simulink model "TFlex_I_FITC"  (R2018a)
settings: Solver=VariableStepAuto  StartTime=0.0  StopTime=10.0  RelTol=1e-3
undefined symbols (not defined in the file): a0, a1, a2, Avout, b, D, DiscIntNeverNeededParam, FB1_offset, h, hyp, I_limit_max, I_limit_min, Kd, Ki, Kp, kp, KTY_p0, KTY_p1, Kuu, LPden, LPnum, Lu, mu_u, Nkeep, R, r, seed, sf, SIGMA, sn, sp_ts, tau_i, tau_p, tau_z, tm, ts, var_u, w
libraries: xpcethercatlib x17, simulink x10, dspindex x6, slrtlib x5, dspfactors x2, dspmtrx3 x2
(part 1 of 2)
settings Model: Creator=wout7  LastModifiedBy=wout7

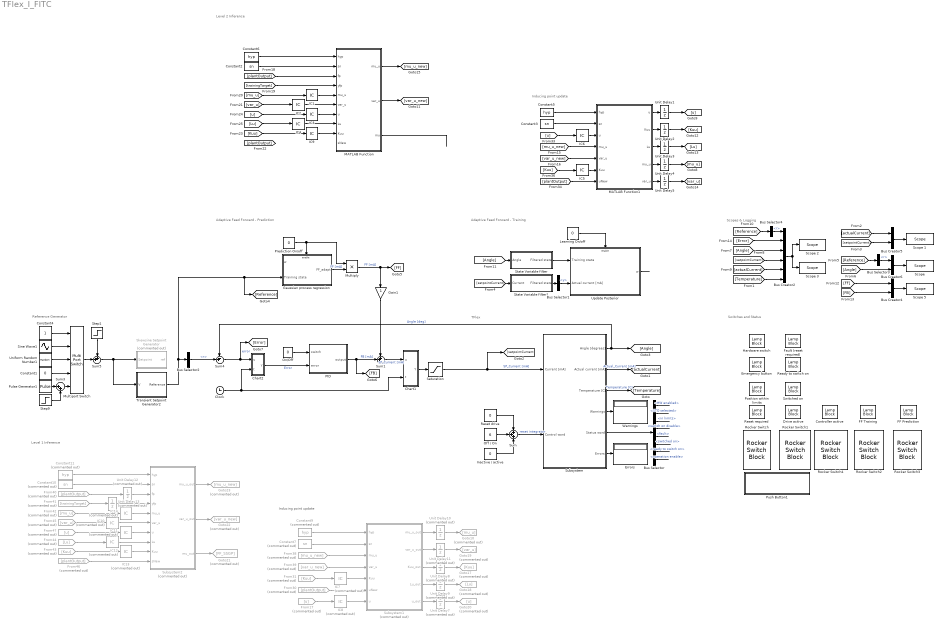
== system TFlex_I_FITC ==
  note: Switches and Status
  note: Adaptive Feed Forward - Prediction
  note: TFlex
  note: Scopes & Logging
  note: Reference Generator
  note: Adaptive Feed Forward - Training
  note: Inducing point update
  note: Inducing point update
  note: Level 2 Inference
  note: Level 1 Inference
  Bus Creator2 : BusCreator  Inputs=6
  Bus Creator4 : BusCreator  Inputs=2
  Bus Creator5 : BusCreator  Inputs=2
  Bus Creator6 : BusCreator  Inputs=2
  Bus Selector : BusSelector  OutputSignals=HW enabled,STO selected,in limits,switch on disable,fault,switched on,ready to switch on,operation enable
  Bus Selector1 : BusSelector  OutputSignals=y
  Bus Selector2 : BusSelector  OutputSignals=r
  Bus Selector3 : BusSelector  OutputSignals=r
  Bus Selector4 : BusSelector  OutputSignals=r
  Chart1 : Stateflow chart  TreatAsAtomicUnit=on
  Chart2 : Stateflow chart  TreatAsAtomicUnit=on
  Clock : Clock
  Constant1 : Constant  Value=0  SampleTime=sp_ts
  Constant10 : Constant  Commented=on  Value=sn  SampleTime=-1
  Constant11 : Constant  Commented=on  Value=hyp  SampleTime=-1
  Constant2 : Constant  Value=sn  SampleTime=-1
  Constant3 : Constant  Value=sn  SampleTime=-1
  Constant4 : Constant  SampleTime=sp_ts
  Constant5 : Constant  Value=hyp  SampleTime=-1
  Constant6 : Constant  Value=hyp  SampleTime=-1
  Constant7 : Constant  Commented=on  Value=sn  SampleTime=-1
  Constant9 : Constant  Commented=on  Value=hyp  SampleTime=-1
  Controller active : LampBlock  WebBlockId=392  LabelPosition=Hide
  Drive active : LampBlock  WebBlockId=394
  Emergency button : LampBlock  WebBlockId=395
  Errors : Display
  FF Prediction : LampBlock  WebBlockId=397  LabelPosition=Hide
  FF Training : LampBlock  WebBlockId=398  LabelPosition=Hide
  Fault (reset required) : LampBlock  WebBlockId=399
  From17 : From  Commented=on  GotoTag=u
  From30 : From  Commented=on  GotoTag=plantOutput
  From31 : From  Commented=on  GotoTag=Kuu
  From38 : From  Commented=on  GotoTag=mu_u_new
  From39 : From  Commented=on  GotoTag=var_u_new
  From40 : From  Commented=on  GotoTag=plantOutput
  From41 : From  Commented=on  GotoTag=trainingTarget
  From42 : From  Commented=on  GotoTag=mu_u
  From43 : From  Commented=on  GotoTag=Kuu
  From44 : From  Commented=on  GotoTag=Lu
  From45 : From  Commented=on  GotoTag=var_u
  From46 : From  Commented=on  GotoTag=plantOutput
  From47 : From  Commented=on  GotoTag=u
  Gain1 : Gain
  Gaussian process regression : Subsystem
  Goto10 : Goto  Commented=on  GotoTag=mu_u
  Goto17 : Goto  Commented=on  GotoTag=Kuu
  Goto18 : Goto  Commented=on  GotoTag=Lu
  Goto19 : Goto  Commented=on  GotoTag=var_u
  Goto20 : Goto  Commented=on  GotoTag=u
  Goto21 : Goto  Commented=on  GotoTag=FF_SSGP
  Goto22 : Goto  Commented=on  GotoTag=var_u_new
  Goto23 : Goto  Commented=on  GotoTag=mu_u_new
  Hardware switch : LampBlock  WebBlockId=462
  IC1 : InitialCondition  Value=mu_u
  IC10 : InitialCondition  Commented=on  Value=var_u
  IC11 : InitialCondition  Commented=on  Value=u
  IC12 : InitialCondition  Commented=on  Value=Lu
  IC13 : InitialCondition  Commented=on  Value=Kuu
  IC14 : InitialCondition  Commented=on  Value=mu_u
  IC2 : InitialCondition  Value=var_u
  IC3 : InitialCondition  Value=u
  IC4 : InitialCondition  Value=Lu
  IC5 : InitialCondition  Value=Kuu
  IC6 : InitialCondition  Value=u
  IC7 : InitialCondition  Commented=on  Value=Kuu
  IC8 : InitialCondition  Commented=on  Value=u
  IC9 : InitialCondition  Value=Kuu
  Inactive / active : Constant  Value=0
  Learning On/off : Constant  Value=0
  MATLAB Function : MATLAB Function  TreatAsAtomicUnit=on
  MATLAB Function1 : MATLAB Function  TreatAsAtomicUnit=on
  Multiply : Product
  Multiport Switch : MultiPortSwitch  Inputs=4
  Off / On : Constant  Value=6
  On/Off : Constant  Value=0
  "PID " : Subsystem
  Position within limits : LampBlock  WebBlockId=527
  Prediction On/off : Constant  Value=0  SampleTime=ts
  Pulse Generator1 : DiscretePulseGenerator  Amplitude=46  SampleTime=sp_ts
  Push Button1 : Subsystem  DialogController=hmiCreateDDGDialog  IsWebBlock=on  mask(MWDashboardBlock){webBlockId=a54107f9-bd11-456c-ac83-5802f3df51ad, webBlockType=pushbutton, ShowInLibBrwoser=on, ShowInitialText=on, HMISrcModelName=TFlex_I_FITC}
      mask prompts: webBlockId "WebBlock Id"; webBlockType "WebBlock Type"; HMISrcModelName "Source Model"
      mask help: SimulinkHMI:dialogs:PushButtonDialogDesc
      mask Help: helpview([docroot '/mapfiles/simulink.map'], 'hmi_push_button')
      mask Display:
      | model = bdroot(gcb);
      | if strcmp(get_param(model,'BlockDiagramType'), 'library')
      |     image([(matlabroot) '/toolbox/simulink/hmi/icons/PushButton.png']);
      | end
  Ready to switch on : LampBlock  WebBlockId=531
  Reset drive : Constant  Value=0
  Reset required : LampBlock  WebBlockId=533
  Rocker Switch : RockerSwitchBlock  WebBlockId=534  LabelPosition=Hide
      settings: Values={{'Off', 'Driver On'}, [6 7]}
  Rocker Switch1 : RockerSwitchBlock  WebBlockId=535  LabelPosition=Hide
      settings: Values={{'Inactive', 'Driver Active'}, [0 8]}
  Rocker Switch2 : RockerSwitchBlock  WebBlockId=536  LabelPosition=Hide
      settings: Values={{'Off', 'Training on'}, [0 1]}
  Rocker Switch3 : RockerSwitchBlock  WebBlockId=537  LabelPosition=Hide
      settings: Values={{'Off', 'Prediction On'}, [0 1]}
  Rocker Switch4 : RockerSwitchBlock  WebBlockId=538  LabelPosition=Hide
      settings: Values={{'Off', 'Controller On'}, [0 1]}
  Saturation : Saturate  UpperLimit=750  LowerLimit=-250/2
  "Scope " : slrtlib/Displays and Logging/Scope   scopeno=1  scopetype=Target  autostart=on  viewmode=Graphical redraw  formatstr='%15.6f'  grid=on  ylimits=[0 ,0]  nosamples=2000  noprepostsamples=0  interleave=1  triggermode=FreeRun  triggersignal=1  trigsignalfromport=off  triggerlevel=0.0  triggerslope=Either  triggerscope=1  triggersample=0  filename=data.dat  mode=Lazy  writesize=512  autorestart=off  dynamicfilemode=off  maxwritefilesize=512*1024^2
  Scope 1 : slrtlib/Displays and Logging/Scope   scopeno=2  scopetype=Target  autostart=on  viewmode=Graphical redraw  formatstr='%15.6f'  grid=on  ylimits=[500,500]  nosamples=250  noprepostsamples=0  interleave=1  triggermode=FreeRun  triggersignal=1  trigsignalfromport=off  triggerlevel=0.0  triggerslope=Either  triggerscope=1  triggersample=0  filename=data.dat  mode=Lazy  writesize=512  autorestart=off  dynamicfilemode=off  maxwritefilesize=512*1024^2
  Scope 2 : slrtlib/Displays and Logging/Scope   scopeno=3  scopetype=Target  autostart=on  viewmode=Numerical  formatstr='%15.6f,%15.6f,%15.6f,%15.0f'  grid=on  ylimits=[500,500]  nosamples=250  noprepostsamples=0  interleave=1  triggermode=FreeRun  triggersignal=1  trigsignalfromport=off  triggerlevel=0.0  triggerslope=Either  triggerscope=1  triggersample=0  filename=data.dat  mode=Lazy  writesize=512  autorestart=off  dynamicfilemode=off  maxwritefilesize=512*1024^2
  Scope 3 : slrtlib/Displays and Logging/Scope   scopeno=4  scopetype=File  autostart=on  viewmode=Graphical redraw  formatstr='%15.6f'  grid=on  ylimits=[0,0]  nosamples=600000  noprepostsamples=0  interleave=1  triggermode=FreeRun  triggersignal=1  trigsignalfromport=off  triggerlevel=0.0  triggerslope=Either  triggerscope=1  triggersample=0  filename=data.dat  mode=Lazy  writesize=512  autorestart=off  dynamicfilemode=off  maxwritefilesize=512*1024^2
  Scope 5 : slrtlib/Displays and Logging/Scope   scopeno=5  scopetype=Target  autostart=on  viewmode=Graphical redraw  formatstr='%15.6f'  grid=on  ylimits=[500,500]  nosamples=250  noprepostsamples=0  interleave=1  triggermode=FreeRun  triggersignal=1  trigsignalfromport=off  triggerlevel=0.0  triggerslope=Either  triggerscope=1  triggersample=0  filename=data.dat  mode=Lazy  writesize=512  autorestart=off  dynamicfilemode=off  maxwritefilesize=512*1024^2
  Sine Wave1 : Sin  Amplitude=15  Frequency=2*pi*2  SampleTime=0
  Skewsine Setpoint Generator : Subsystem  Commented=on
  State Variable filter : Subsystem
  State Variable filter1 : Subsystem
  Step1 : Step  Time=20  Before=-23  After=0  SampleTime=0
  Step9 : Step  Time=0  After=-24  SampleTime=sp_ts
  Subsystem : Subsystem
  Subsystem1 : Subsystem  Commented=on
  Subsystem2 : Subsystem  Commented=on
  Sum : Sum  Inputs=+++
  Sum1 : Sum  Inputs=++|
  Sum3 : Sum  Inputs=|++
  Sum4 : Sum  Inputs=-+|
  Sum5 : Sum  Inputs=++|
  Switched on : LampBlock  WebBlockId=680
  Transient Setpoint Generator2 : Subsystem
  Uniform Random Number1 : UniformRandomNumber  Seed=seed  SampleTime=sp_ts
  Unit Delay{1..5} (5 alike) : UnitDelay  SampleTime=-1
  Unit Delay{7..13} (7 alike) : UnitDelay  Commented=on  SampleTime=-1
  Update Posterior : Subsystem
  Warnings : Display
  wires:
  Bus Selector/5 -> ?  "<fault>"
  Bus Selector/8 -> ?  "<operation enable>"
  Bus Selector/7 -> ?  "<ready to switch on>"
  Bus Selector/3 -> ?  "<in limits>"
  Update Posterior/1(w) -> ?
  Subsystem/5(Status word) -> Bus Selector/1
  ? -> Gaussian process regression/1(w)
  Subsystem/1(Angle [degrees]) -> [Angle], Sum4/1  "Angle [deg]"
  Subsystem/6(Errors) -> Errors/1
  Subsystem/2(Actual current [mA]) -> [actualCurrent]  "Actual_Current [mA]"
  Pulse Generator1/1 -> Sum3/1
  Bus Selector/1 -> ?  "<HW enabled>"
  Step9/1 -> Sum3/2
  Gaussian process regression/1(FF_adapt) -> Multiply/2  "FF [mA]"
  [FB] -> Bus Creator4/2
  State Variable filter/1(Filtered state) -> Update Posterior/1(Training state)
  Reset drive/1 -> Sum/1
  Sum3/1 -> Multiport Switch/5
  Constant1/1 -> Multiport Switch/4
  Bus Selector/2 -> ?  "<STO selected>"
  Multiply/1 -> Gain1/1, [FF]  "FF [mA]"
  Bus Selector3/1 -> Bus Creator6/1  "<r>"
  Step1/1 -> Sum5/1
  Bus Creator6/1 -> "Scope "/1
  Saturation/1 -> [setpointCurrent], Subsystem/1(Current [mA])  "SP_Current [mA]"
  Subsystem/3(Temperature [C]) -> [Temperature]  "Temperature [C]"
  Sum/1 -> Subsystem/2(Control word)  "reset integrator"
  Bus Selector4/1 -> Bus Creator2/1  "<r>"
  Chart2/1(Y) -> "PID "/2(error)  "Error"
  Bus Creator5/1 -> Scope 1/1
  [Error] -> Bus Creator2/2
  [setpointCurrent] -> Bus Creator2/4
  Bus Creator4/1 -> Scope 5/1
  State Variable filter1/1(Filtered state) -> Bus Selector1/1
  Bus Selector/4 -> ?  "<switch on disable>"
  [Angle] -> Bus Creator6/2
  Chart1/1(Y) -> Saturation/1
  "PID "/1(output) -> [FB], Sum1/2  "FB [mA]"
  [FF] -> Bus Creator4/1
  [setpointCurrent] -> State Variable filter1/1(Current)
  [actualCurrent] -> Bus Creator5/1
  Sine Wave1/1 -> Multiport Switch/2
  [actualCurrent] -> Bus Creator2/5
  Subsystem/4(Warnings) -> Warnings/1
  [setpointCurrent] -> Bus Creator5/2
  Gain1/1 -> Sum1/1
  Sum1/1 -> Chart1/1(u)  "SP_Current [mA]"
  [Reference] -> Bus Selector3/1
  [Temperature] -> Bus Creator2/6
  Sum5/1 -> Skewsine Setpoint Generator/1(Setpoint), Transient Setpoint Generator2/1(V)
  [Reference] -> Bus Selector4/1
  Bus Selector2/1 -> Sum4/2  "<r>"
  Bus Selector1/1 -> Update Posterior/2("Actual current [mA] ")  "<y>"
  Inactive / active/1 -> Sum/3
  [Angle] -> State Variable filter/1(Angle)
  Uniform Random Number1/1 -> Multiport Switch/3
  Bus Creator2/1 -> Scope 2/1, Scope 3/1
  Prediction On/off/1 -> Gaussian process regression/Enable, Multiply/1
  Multiport Switch/1 -> Sum5/2
  Clock/1 -> Chart2/2(t), Chart1/2(t)
  Transient Setpoint Generator2/1(Reference) -> Gaussian process regression/2(Training state), [Reference], Bus Selector2/1
  Sum4/1 -> [Error], Chart2/1(u)  "error"
  Learning On/off/1 -> Update Posterior/Enable
  [Angle] -> Bus Creator2/3
  Off / On/1 -> Sum/2
  Constant4/1 -> Multiport Switch/1
  Bus Selector/6 -> ?  "<switched on>"
  On/Off/1 -> "PID "/1(switch)
  Constant3/1 -> MATLAB Function1/2(sn)
  MATLAB Function1/4(mu_u) -> Unit Delay4/1
  [u] -> IC6/1
  [plantOutput] -> MATLAB Function1/7(uNew)
  [Kuu] -> IC5/1
  IC6/1 -> MATLAB Function1/3("u ")
  Unit Delay3/1 -> [Lu]
  [var_u_new] -> MATLAB Function1/5("var_u ")
  MATLAB Function1/5(var_u) -> Unit Delay5/1
  Constant5/1 -> MATLAB Function1/1(hyp)
  Unit Delay4/1 -> [mu_u]
  MATLAB Function1/2(Kuu) -> Unit Delay2/1
  [mu_u_new] -> MATLAB Function1/4("mu_u ")
  MATLAB Function1/1(u) -> Unit Delay1/1
  IC5/1 -> MATLAB Function1/6("Kuu ")
  Unit Delay5/1 -> [var_u]
  MATLAB Function1/3(Lu) -> Unit Delay3/1
  Unit Delay1/1 -> [u]
  Unit Delay2/1 -> [Kuu]
  Unit Delay9/1 -> Goto18/1
  From31/1 -> IC7/1
  Unit Delay7/1 -> Goto20/1
  Subsystem1/5(u_out) -> Unit Delay7/1
  From17/1 -> IC8/1
  From39/1 -> Subsystem1/4(var_u)
  IC7/1 -> Subsystem1/5(Kuu)
  From38/1 -> Subsystem1/3(mu_u)
  Subsystem1/4(Lu_out) -> Unit Delay9/1
  Subsystem1/3(Kuu_out) -> Unit Delay8/1
  Unit Delay11/1 -> Goto19/1
  Constant9/1 -> Subsystem1/1(hyp)
  Subsystem1/2(var_u_out) -> Unit Delay11/1
  Unit Delay10/1 -> Goto10/1
  From30/1 -> Subsystem1/6(uNew)
  Unit Delay8/1 -> Goto17/1
  Constant7/1 -> Subsystem1/2(sn)
  Subsystem1/1(mu_u_out) -> Unit Delay10/1
  IC8/1 -> Subsystem1/7(u)
  [plantOutput] -> MATLAB Function/3(fp)
  [trainingTarget] -> MATLAB Function/4(yfp)
  IC4/1 -> MATLAB Function/8(Lu)
  IC1/1 -> MATLAB Function/5("mu_u ")
  [Kuu] -> IC9/1
  [var_u] -> IC2/1
  [u] -> IC3/1
  [Lu] -> IC4/1
  Constant2/1 -> MATLAB Function/2(sn)
  [mu_u] -> IC1/1
  IC9/1 -> MATLAB Function/9(Kuu)
  MATLAB Function/1(mu_u) -> [mu_u_new]
  ? -> MATLAB Function/10(sNew)
  MATLAB Function/2(var_u) -> [var_u_new]
  IC2/1 -> MATLAB Function/6("var_u ")
  IC3/1 -> MATLAB Function/7(u)
  Constant6/1 -> MATLAB Function/1(hyp)
  MATLAB Function/3(mu) -> ?
  From44/1 -> IC12/1
  From47/1 -> IC11/1
  Constant11/1 -> Subsystem2/1(hyp)
  Subsystem2/2(var_u_out) -> Goto22/1
  IC12/1 -> Subsystem2/8(Lu)
  Unit Delay12/1 -> Subsystem2/3(fp)
  IC11/1 -> Subsystem2/7(u)
  IC13/1 -> Subsystem2/9(Kuu)
  Unit Delay13/1 -> Subsystem2/4(yfp)
  From40/1 -> Unit Delay12/1
  IC14/1 -> Subsystem2/5(mu_u)
  From46/1 -> Subsystem2/10(sNew)
  Subsystem2/3(mu_out) -> Goto21/1
  From43/1 -> IC13/1
  Subsystem2/1(mu_u_out) -> Goto23/1
  From45/1 -> IC10/1
  From42/1 -> IC14/1
  From41/1 -> Unit Delay13/1
  Constant10/1 -> Subsystem2/2(sn)
  IC10/1 -> Subsystem2/6(var_u)

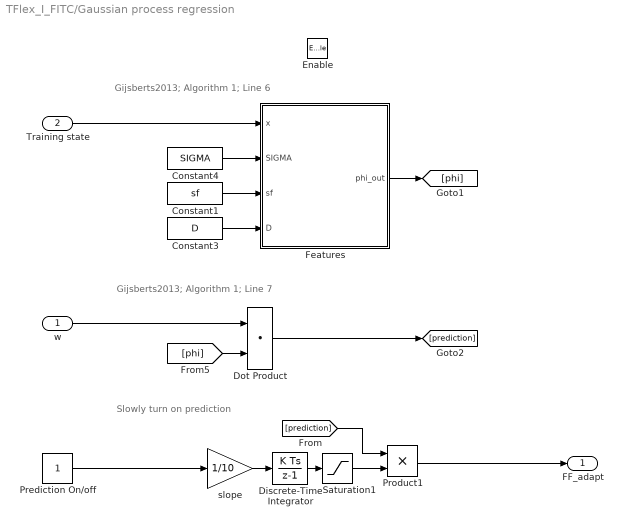
== system TFlex_I_FITC/Gaussian process regression ==
  note: Gijsberts2013; Algorithm 1; Line 7
  note: Gijsberts2013; Algorithm 1; Line 6
  note: Slowly turn on prediction
  w : Inport
  Training state : Inport  Port=2
  Enable : EnablePort  StatesWhenEnabling=reset
  Constant1 : Constant  Value=sf  VectorParams1D=off
  Constant3 : Constant  Value=D  VectorParams1D=off
  Constant4 : Constant  Value=SIGMA  VectorParams1D=off
  Discrete-Time Integrator : DiscreteIntegrator  SampleTime=-1  ICPrevOutput=DiscIntNeverNeededParam  ICPrevScaledInput=DiscIntNeverNeededParam
  Dot Product : DotProduct  OutDataTypeStr=Inherit: Inherit via internal rule
  Features : Subsystem
  Prediction On/off : Constant
  Product1 : Product
  Saturation1 : Saturate  UpperLimit=1  LowerLimit=0
  slope : Gain  Gain=1/10
  FF_adapt : Outport  SampleTime=ts
  wires:
  w/1 -> Dot Product/1
  [phi] -> Dot Product/2
  Product1/1 -> FF_adapt/1
  slope/1 -> Discrete-Time Integrator/1
  Prediction On/off/1 -> slope/1
  Discrete-Time Integrator/1 -> Saturation1/1
  Dot Product/1 -> [prediction]
  Constant4/1 -> Features/2(SIGMA)
  Training state/1 -> Features/1(x)
  Features/1(phi_out) -> [phi]
  Constant3/1 -> Features/4(D)
  Constant1/1 -> Features/3(sf)
  Saturation1/1 -> Product1/2
  [prediction] -> Product1/1

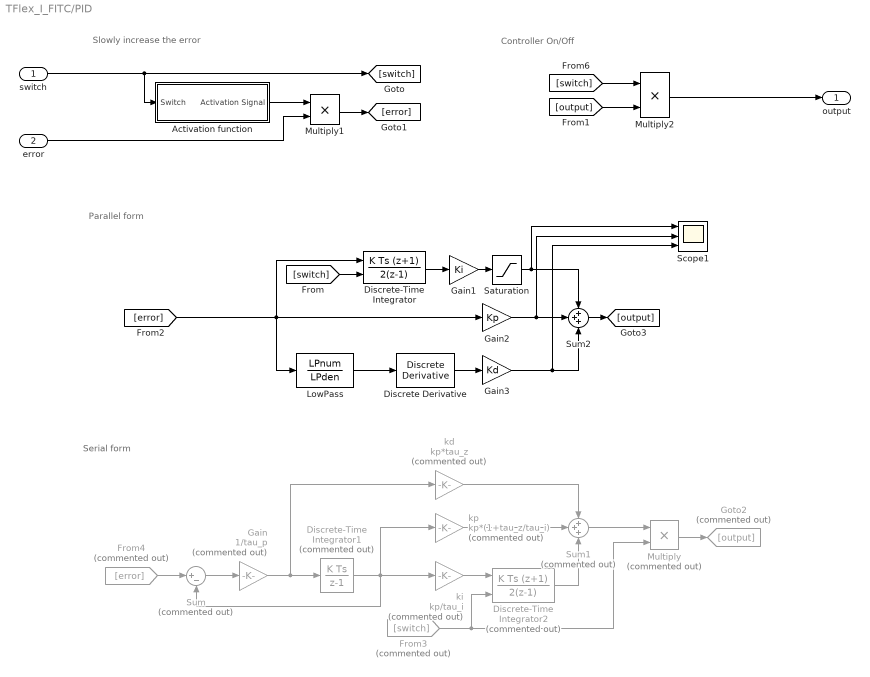
== system TFlex_I_FITC/PID  ==
  note: Controller On/Off
  note: Slowly increase the error
  note: Serial form
  note: Parallel form
  switch : Inport  SampleTime=ts
  error : Inport  Port=2
  Activation function : Subsystem
  Discrete Derivative : simulink/Discrete/Discrete Derivative  gainval=1.0  ICPrevScaledInput=0.0  OutMin=[]  OutMax=[]  OutDataType=fixdt(1, 16)  OutScaling=2^-10  DoSatur=off
  Discrete-Time Integrator : DiscreteIntegrator  IntegratorMethod=Integration: Trapezoidal  ExternalReset=either  SampleTime=ts  LimitOutput=on  UpperSaturationLimit=I_limit_max  LowerSaturationLimit=I_limit_min  ICPrevOutput=DiscIntNeverNeededParam  ICPrevScaledInput=DiscIntNeverNeededParam
  Discrete-Time Integrator1 : DiscreteIntegrator  Commented=on  SampleTime=-1  ICPrevOutput=DiscIntNeverNeededParam  ICPrevScaledInput=DiscIntNeverNeededParam
  Discrete-Time Integrator2 : DiscreteIntegrator  Commented=on  IntegratorMethod=Integration: Trapezoidal  ExternalReset=rising  SampleTime=ts  LimitOutput=on  UpperSaturationLimit=I_limit_max  LowerSaturationLimit=I_limit_min  ICPrevOutput=DiscIntNeverNeededParam  ICPrevScaledInput=DiscIntNeverNeededParam
  From3 : From  Commented=on  GotoTag=switch
  From4 : From  Commented=on  GotoTag=error
  Gain : Gain  Commented=on  Gain=1/tau_p
  Gain1 : Gain  Gain=Ki
  Gain2 : Gain  Gain=Kp
  Gain3 : Gain  Gain=Kd
  Goto2 : Goto  Commented=on  GotoTag=output
  LowPass : DiscreteTransferFcn  Numerator=LPnum  Denominator=LPden
  Multiply : Product  Commented=on
  Multiply1 : Product
  Multiply2 : Product
  Saturation : Saturate  UpperLimit=I_limit_max  LowerLimit=I_limit_min
  Scope1 : Scope  NumInputPorts=3
  Sum : Sum  Commented=on  Inputs=|+-
  Sum1 : Sum  Commented=on  Inputs=+++
  Sum2 : Sum  Inputs=+++
  kd : Gain  Commented=on  Gain=kp*tau_z
  ki : Gain  Commented=on  Gain=kp/tau_i
  kp : Gain  Commented=on  Gain=kp*(1+tau_z/tau_i)
  output : Outport
  wires:
  LowPass/1 -> Discrete Derivative/1
  [error] -> Discrete-Time Integrator/1, Gain2/1, LowPass/1
  Discrete-Time Integrator/1 -> Gain1/1
  Gain2/1 -> Scope1/2, Sum2/2
  Gain3/1 -> Scope1/3, Sum2/3
  Sum2/1 -> [output]
  Sum/1 -> Gain/1
  Gain/1 -> Discrete-Time Integrator1/1, kd/1
  ki/1 -> Discrete-Time Integrator2/1
  Discrete-Time Integrator1/1 -> kp/1, ki/1, Sum/2
  kp/1 -> Sum1/2
  kd/1 -> Sum1/1
  Discrete-Time Integrator2/1 -> Sum1/3
  Discrete Derivative/1 -> Gain3/1
  From4/1 -> Sum/1
  Sum1/1 -> Multiply/1
  From3/1 -> Discrete-Time Integrator2/2, Multiply/2
  Multiply/1 -> Goto2/1
  switch/1 -> [switch], Activation function/1(Switch)
  error/1 -> Multiply1/2
  [output] -> Multiply2/2
  [switch] -> Discrete-Time Integrator/2
  Multiply1/1 -> [error]
  [switch] -> Multiply2/1
  Multiply2/1 -> output/1
  Saturation/1 -> Sum2/1, Scope1/1
  Gain1/1 -> Saturation/1
  Activation function/1(Activation Signal) -> Multiply1/1

== system TFlex_I_FITC/Push Button1 ==

== system TFlex_I_FITC/Skewsine Setpoint Generator ==
  Setpoint : Inport
  Bus Creator : BusCreator  Inputs=3
  Delay : Delay  Commented=through  DelayLength=1  InitialCondition=0
  Subsystem : Subsystem
  ref : Outport
  wires:
  Subsystem/3(r_ddot) -> Bus Creator/3  "r_ddot"
  Bus Creator/1 -> ref/1
  Setpoint/1 -> Delay/1
  Subsystem/2(r_dot) -> Bus Creator/2  "r_dot"
  Subsystem/1(r) -> Bus Creator/1  "r"
  Delay/1 -> Subsystem/1(setpoint)

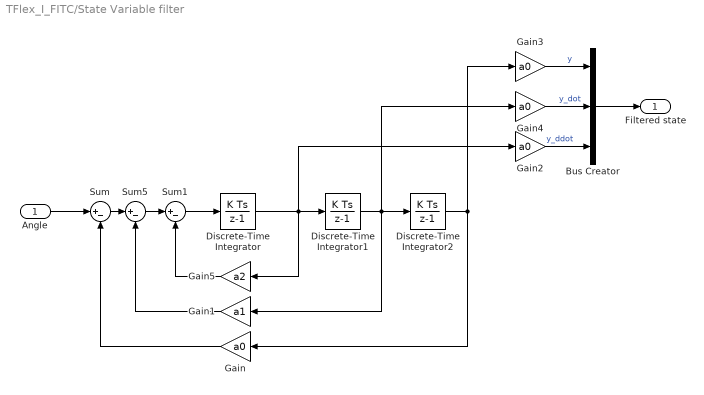
== system TFlex_I_FITC/State Variable filter ==
  Angle : Inport
  Bus Creator : BusCreator  Inputs=3
  Discrete-Time Integrator : DiscreteIntegrator  SampleTime=-1  ICPrevOutput=DiscIntNeverNeededParam  ICPrevScaledInput=DiscIntNeverNeededParam
  Discrete-Time Integrator1 : DiscreteIntegrator  SampleTime=-1  ICPrevOutput=DiscIntNeverNeededParam  ICPrevScaledInput=DiscIntNeverNeededParam
  Discrete-Time Integrator2 : DiscreteIntegrator  SampleTime=-1  ICPrevOutput=DiscIntNeverNeededParam  ICPrevScaledInput=DiscIntNeverNeededParam
  Gain{,2..4} (4 alike) : Gain  Gain=a0
  Gain1 : Gain  Gain=a1
  Gain5 : Gain  Gain=a2
  Sum : Sum  Inputs=|+-
  Sum1 : Sum  Inputs=|+-
  Sum5 : Sum  Inputs=|+-
  Filtered state : Outport
  wires:
  Bus Creator/1 -> Filtered state/1
  Angle/1 -> Sum/1
  Sum/1 -> Sum5/1
  Gain/1 -> Sum/2
  Gain1/1 -> Sum5/2
  Gain3/1 -> Bus Creator/1  "y"
  Gain2/1 -> Bus Creator/3  "y_ddot"
  Gain4/1 -> Bus Creator/2  "y_dot"
  Gain5/1 -> Sum1/2
  Sum5/1 -> Sum1/1
  Sum1/1 -> Discrete-Time Integrator/1
  Discrete-Time Integrator/1 -> Discrete-Time Integrator1/1, Gain2/1, Gain5/1
  Discrete-Time Integrator1/1 -> Discrete-Time Integrator2/1, Gain4/1, Gain1/1
  Discrete-Time Integrator2/1 -> Gain3/1, Gain/1

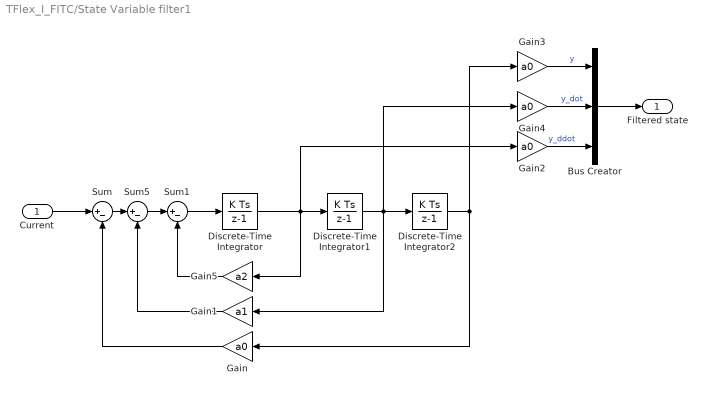
== system TFlex_I_FITC/State Variable filter1 ==
  Current : Inport
  Bus Creator : BusCreator  Inputs=3
  Discrete-Time Integrator : DiscreteIntegrator  SampleTime=-1  ICPrevOutput=DiscIntNeverNeededParam  ICPrevScaledInput=DiscIntNeverNeededParam
  Discrete-Time Integrator1 : DiscreteIntegrator  SampleTime=-1  ICPrevOutput=DiscIntNeverNeededParam  ICPrevScaledInput=DiscIntNeverNeededParam
  Discrete-Time Integrator2 : DiscreteIntegrator  SampleTime=-1  ICPrevOutput=DiscIntNeverNeededParam  ICPrevScaledInput=DiscIntNeverNeededParam
  Gain{,2..4} (4 alike) : Gain  Gain=a0
  Gain1 : Gain  Gain=a1
  Gain5 : Gain  Gain=a2
  Sum : Sum  Inputs=|+-
  Sum1 : Sum  Inputs=|+-
  Sum5 : Sum  Inputs=|+-
  Filtered state : Outport
  wires:
  Bus Creator/1 -> Filtered state/1
  Current/1 -> Sum/1
  Sum/1 -> Sum5/1
  Gain/1 -> Sum/2
  Gain1/1 -> Sum5/2
  Gain3/1 -> Bus Creator/1  "y"
  Gain2/1 -> Bus Creator/3  "y_ddot"
  Gain4/1 -> Bus Creator/2  "y_dot"
  Gain5/1 -> Sum1/2
  Sum5/1 -> Sum1/1
  Sum1/1 -> Discrete-Time Integrator/1
  Discrete-Time Integrator/1 -> Discrete-Time Integrator1/1, Gain2/1, Gain5/1
  Discrete-Time Integrator1/1 -> Discrete-Time Integrator2/1, Gain4/1, Gain1/1
  Discrete-Time Integrator2/1 -> Gain3/1, Gain/1

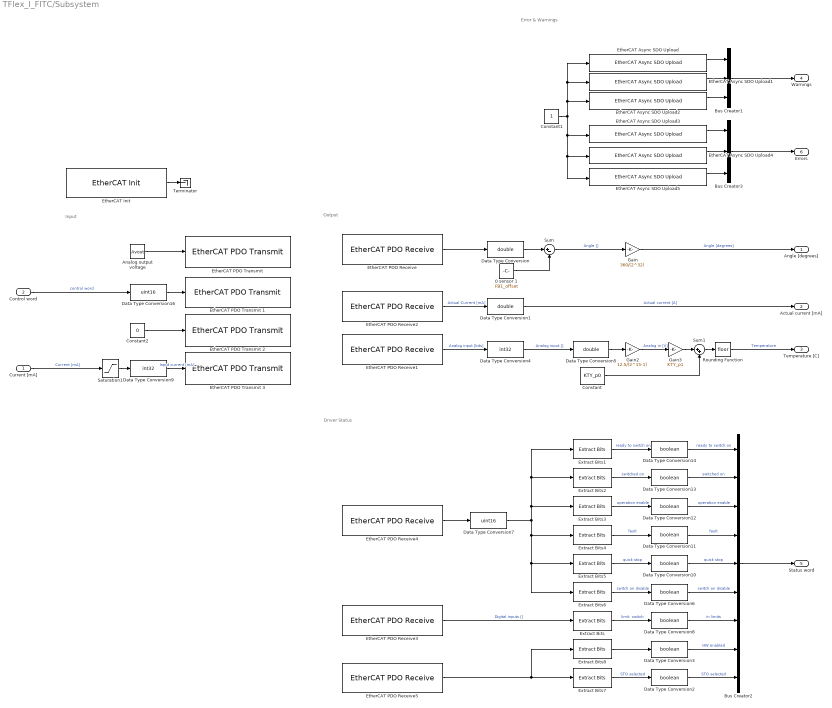
== system TFlex_I_FITC/Subsystem ==
  note: Output
  note: Error & Warnings
  note: Driver Status
  note: Input
  Current [mA] : Inport
  Control word : Inport  Port=2
  0 sensor 1 : Constant  Value=FB1_offset
  Analog output voltage : Constant  Value=Avout  OutDataTypeStr=int16
  Bus Creator1 : BusCreator  Inputs=3
  Bus Creator2 : BusCreator  Inputs=9
  Bus Creator3 : BusCreator  Inputs=3
  Constant : Constant  Value=KTY_p0
  Constant1 : Constant  OutDataTypeStr=int32
  Constant2 : Constant  Value=0  OutDataTypeStr=uint32
  Data Type Conversion : DataTypeConversion  OutDataTypeStr=double
  Data Type Conversion1 : DataTypeConversion  OutDataTypeStr=double
  Data Type Conversion{2..3,6,8,10..14} (9 alike) : DataTypeConversion  OutDataTypeStr=boolean
  Data Type Conversion16 : DataTypeConversion  OutDataTypeStr=uint16
  Data Type Conversion4 : DataTypeConversion  OutDataTypeStr=int32
  Data Type Conversion5 : DataTypeConversion  OutDataTypeStr=double
  Data Type Conversion7 : DataTypeConversion  OutDataTypeStr=uint16  RndMeth=Round
  Data Type Conversion9 : DataTypeConversion  OutDataTypeStr=int32
  EtherCAT Async SDO Upload : xpcethercatlib/EtherCAT Async SDO Upload  index=8192  subIndex=1  sig_type=uint32  sig_dim=1  device_id=0  slave_name=Drive 1 (AKD)  sample_time=1  slave_addr=1001  selected_slave=Term 1 (EK1100)  timeout=500  slave_found=1
      settings: SourceProductName=Simulink Real-Time  SourceProductBaseCode=XP
  EtherCAT Async SDO Upload1 : xpcethercatlib/EtherCAT Async SDO Upload  index=8192  subIndex=2  sig_type=uint32  sig_dim=1  device_id=0  slave_name=Drive 1 (AKD)  sample_time=1  slave_addr=1001  selected_slave=Term 1 (EK1100)  timeout=500  slave_found=1
      settings: SourceProductName=Simulink Real-Time  SourceProductBaseCode=XP
  EtherCAT Async SDO Upload2 : xpcethercatlib/EtherCAT Async SDO Upload  index=8192  subIndex=3  sig_type=uint32  sig_dim=1  device_id=0  slave_name=Drive 1 (AKD)  sample_time=1  slave_addr=1001  selected_slave=Term 1 (EK1100)  timeout=500  slave_found=1
      settings: SourceProductName=Simulink Real-Time  SourceProductBaseCode=XP
  EtherCAT Async SDO Upload3 : xpcethercatlib/EtherCAT Async SDO Upload  index=8193  subIndex=1  sig_type=uint32  sig_dim=1  device_id=0  slave_name=Drive 1 (AKD)  sample_time=1  slave_addr=1001  selected_slave=Term 1 (EK1100)  timeout=500  slave_found=1
      settings: SourceProductName=Simulink Real-Time  SourceProductBaseCode=XP
  EtherCAT Async SDO Upload4 : xpcethercatlib/EtherCAT Async SDO Upload  index=8193  subIndex=2  sig_type=uint32  sig_dim=1  device_id=0  slave_name=Drive 1 (AKD)  sample_time=1  slave_addr=1001  selected_slave=Term 1 (EK1100)  timeout=500  slave_found=1
      settings: SourceProductName=Simulink Real-Time  SourceProductBaseCode=XP
  EtherCAT Async SDO Upload5 : xpcethercatlib/EtherCAT Async SDO Upload  index=8193  subIndex=3  sig_type=uint32  sig_dim=1  device_id=0  slave_name=Drive 1 (AKD)  sample_time=1  slave_addr=1001  selected_slave=Term 1 (EK1100)  timeout=500  slave_found=1
      settings: SourceProductName=Simulink Real-Time  SourceProductBaseCode=XP
  "EtherCAT Init " : xpcethercatlib/EtherCAT Init   Priority=0  config_file=C:\Users\wout7\Documents\GitHub\Inverse_dynamics_learning\TargetPC\Tflex PID 17-5-2019\custom_pdo_eni3.xml  device_id=1  pci_bus=13  pci_slot=0  pci_function=0  dctuning=0  enaDebug=off  enaDC=on  errLink=off  masterDbg=off  stateChgDbg=off  baseClock=off  masterCfg=off  logFile='c:\dbglog.txt'  sample_time=0.001000  DCMode=2
      settings: SourceProductName=Simulink Real-Time  SourceProductBaseCode=XP
  EtherCAT PDO Receive : xpcethercatlib/EtherCAT PDO Receive  Priority=2  sig_name=Drive 1 (AKD).TPDO mapping parameter 3.Position actual internal value  sig_offset=624  sig_type=int32  type_size=32  sig_dim=1  device_id=0  sample_time=0.001000
      settings: SourceProductName=Simulink Real-Time  SourceProductBaseCode=XP
  EtherCAT PDO Receive1 : xpcethercatlib/EtherCAT PDO Receive  Priority=2  sig_name=Drive 1 (AKD).TPDO mapping parameter 1.AOUT_INPUT_VALUE  sig_offset=480  sig_type=int16  type_size=16  sig_dim=1  device_id=0  sample_time=0.001
      settings: SourceProductName=Simulink Real-Time  SourceProductBaseCode=XP
  EtherCAT PDO Receive2 : xpcethercatlib/EtherCAT PDO Receive  Priority=2  sig_name=Drive 1 (AKD).TPDO mapping parameter 2.Current actual value  sig_offset=528  sig_type=int32  type_size=32  sig_dim=1  device_id=0  sample_time=0.001000
      settings: SourceProductName=Simulink Real-Time  SourceProductBaseCode=XP
  EtherCAT PDO Receive3 : xpcethercatlib/EtherCAT PDO Receive  Priority=2  sig_name=Drive 1 (AKD).TPDO mapping parameter 1.Digital inputs  sig_offset=496  sig_type=uint32  type_size=32  sig_dim=1  device_id=0  sample_time=0.001000
      settings: SourceProductName=Simulink Real-Time  SourceProductBaseCode=XP
  EtherCAT PDO Receive4 : xpcethercatlib/EtherCAT PDO Receive  Priority=2  sig_name=Drive 1 (AKD).TPDO mapping parameter 1.Statusword  sig_offset=464  sig_type=uint16  type_size=16  sig_dim=1  device_id=0  sample_time=0.001
      settings: SourceProductName=Simulink Real-Time  SourceProductBaseCode=XP
  EtherCAT PDO Receive5 : xpcethercatlib/EtherCAT PDO Receive  Priority=2  sig_name=Drive 1 (AKD).TPDO mapping parameter 3.Manufacturer status register  sig_offset=592  sig_type=uint32  type_size=32  sig_dim=1  device_id=0  sample_time=0.001000
      settings: SourceProductName=Simulink Real-Time  SourceProductBaseCode=XP
  "EtherCAT PDO Transmit " : xpcethercatlib/EtherCAT PDO Transmit   Priority=3  sig_name=Drive 1 (AKD).RPDO mapping parameter 1.AOUT.VALUE write  sig_offset=480  sig_type=int16  type_size=16  sig_dim=1  device_id=0  sample_time=0.001000
      settings: SourceProductName=Simulink Real-Time  SourceProductBaseCode=XP
  EtherCAT PDO Transmit 1 : xpcethercatlib/EtherCAT PDO Transmit   Priority=3  sig_name=Drive 1 (AKD).RPDO mapping parameter 1.Controlword  sig_offset=464  sig_type=uint16  type_size=16  sig_dim=1  device_id=0  sample_time=0.001000
      settings: SourceProductName=Simulink Real-Time  SourceProductBaseCode=XP
  EtherCAT PDO Transmit 2 : xpcethercatlib/EtherCAT PDO Transmit   Priority=3  sig_name=Drive 1 (AKD).RPDO mapping parameter 1.Physical outputs  sig_offset=496  sig_type=uint32  type_size=32  sig_dim=1  device_id=0  sample_time=0.001000
      settings: SourceProductName=Simulink Real-Time  SourceProductBaseCode=XP
  EtherCAT PDO Transmit 3 : xpcethercatlib/EtherCAT PDO Transmit   Priority=3  sig_name=Drive 1 (AKD).RPDO mapping parameter 2.Target current  sig_offset=528  sig_type=int32  type_size=32  sig_dim=1  device_id=0  sample_time=0.001000
      settings: SourceProductName=Simulink Real-Time  SourceProductBaseCode=XP
  Extract Bits : simulink/Logic and Bit Operations/Extract Bits  bitsToExtract=Range of bits  numBits=8  bitIdxRange=[16]  outScalingMode=Treat bit field as an integer
      settings: SourceProductName=Simulink
  Extract Bits1 : simulink/Logic and Bit Operations/Extract Bits  bitsToExtract=Range of bits  numBits=8  bitIdxRange=[0]  outScalingMode=Treat bit field as an integer
      settings: SourceProductName=Simulink
  Extract Bits2 : simulink/Logic and Bit Operations/Extract Bits  bitsToExtract=Range of bits  numBits=8  bitIdxRange=[1]  outScalingMode=Treat bit field as an integer
      settings: SourceProductName=Simulink
  Extract Bits3 : simulink/Logic and Bit Operations/Extract Bits  bitsToExtract=Range of bits  numBits=8  bitIdxRange=[2]  outScalingMode=Treat bit field as an integer
      settings: SourceProductName=Simulink
  Extract Bits4 : simulink/Logic and Bit Operations/Extract Bits  bitsToExtract=Range of bits  numBits=8  bitIdxRange=[3]  outScalingMode=Treat bit field as an integer
      settings: SourceProductName=Simulink
  Extract Bits5 : simulink/Logic and Bit Operations/Extract Bits  bitsToExtract=Range of bits  numBits=8  bitIdxRange=[5]  outScalingMode=Treat bit field as an integer
      settings: SourceProductName=Simulink
  Extract Bits6 : simulink/Logic and Bit Operations/Extract Bits  bitsToExtract=Range of bits  numBits=8  bitIdxRange=[6]  outScalingMode=Treat bit field as an integer
      settings: SourceProductName=Simulink
  Extract Bits7 : simulink/Logic and Bit Operations/Extract Bits  bitsToExtract=Range of bits  numBits=8  bitIdxRange=[13]  outScalingMode=Treat bit field as an integer
      settings: SourceProductName=Simulink
  Extract Bits8 : simulink/Logic and Bit Operations/Extract Bits  bitsToExtract=Range of bits  numBits=8  bitIdxRange=[29]  outScalingMode=Treat bit field as an integer
      settings: SourceProductName=Simulink
  Gain : Gain  Gain=360/(2^32)
  Gain2 : Gain  Gain=12.5/(2^15-1)
  Gain3 : Gain  Gain=KTY_p1
  Rounding Function : Rounding
  Saturation1 : Saturate  UpperLimit=I_limit_max  LowerLimit=I_limit_min
  Sum : Sum  Inputs=|+-
  Sum1 : Sum  Inputs=|++  OutDataTypeStr=double
  Terminator : Terminator
  Angle [degrees] : Outport
  Actual current [mA] : Outport  Port=2
  Temperature [C] : Outport  Port=3
  Warnings : Outport  Port=4
  Status word : Outport  Port=5
  Errors : Outport  Port=6
  wires:
  Data Type Conversion/1 -> Sum/1
  Data Type Conversion9/1 -> EtherCAT PDO Transmit 3/1  "Input current [mA]"
  Bus Creator2/1 -> Status word/1
  0 sensor 1/1 -> Sum/2
  Data Type Conversion1/1 -> Actual current [mA]/1  "Actual current [A]"
  Data Type Conversion7/1 -> Extract Bits4/1, Extract Bits5/1, Extract Bits6/1, Extract Bits1/1, Extract Bits2/1, Extract Bits3/1
  EtherCAT PDO Receive4/1 -> Data Type Conversion7/1
  EtherCAT PDO Receive2/1 -> Data Type Conversion1/1  "Actual Current [mA]"
  Data Type Conversion4/1 -> Data Type Conversion5/1  "Analog input []"
  EtherCAT PDO Receive/1 -> Data Type Conversion/1
  Gain/1 -> Angle [degrees]/1  "Angle [degrees]"
  EtherCAT PDO Receive5/1 -> Extract Bits8/1, Extract Bits7/1
  EtherCAT PDO Receive1/1 -> Data Type Conversion4/1  "Analog input [bits]"
  Sum/1 -> Gain/1  "Angle []"
  Extract Bits8/1 -> Data Type Conversion3/1
  Extract Bits6/1 -> Data Type Conversion6/1  "switch on disable"
  Extract Bits/1 -> Data Type Conversion8/1  "limit  switch"
  Extract Bits3/1 -> Data Type Conversion12/1  "operation enable"
  Extract Bits2/1 -> Data Type Conversion13/1  "switched on"
  Extract Bits4/1 -> Data Type Conversion11/1  "fault"
  Extract Bits5/1 -> Data Type Conversion10/1  "quick stop"
  Constant2/1 -> EtherCAT PDO Transmit 2/1
  Extract Bits1/1 -> Data Type Conversion14/1  "ready to switch on"
  EtherCAT PDO Receive3/1 -> Extract Bits/1  "Digital inputs []"
  Extract Bits7/1 -> Data Type Conversion2/1  "STO selected"
  Data Type Conversion16/1 -> EtherCAT PDO Transmit 1/1
  "EtherCAT Init "/1 -> Terminator/1
  Data Type Conversion5/1 -> Gain2/1
  Analog output voltage/1 -> "EtherCAT PDO Transmit "/1
  Gain2/1 -> Gain3/1  "Analog in [V]"
  Sum1/1 -> Rounding Function/1
  Rounding Function/1 -> Temperature [C]/1  "Temperature"
  EtherCAT Async SDO Upload/1 -> Bus Creator1/1
  Bus Creator1/1 -> Warnings/1
  Constant1/1 -> EtherCAT Async SDO Upload5/1, EtherCAT Async SDO Upload4/1, EtherCAT Async SDO Upload3/1, EtherCAT Async SDO Upload/1, EtherCAT Async SDO Upload1/1, EtherCAT Async SDO Upload2/1
  EtherCAT Async SDO Upload1/1 -> Bus Creator1/2
  EtherCAT Async SDO Upload2/1 -> Bus Creator1/3
  EtherCAT Async SDO Upload3/1 -> Bus Creator3/1
  EtherCAT Async SDO Upload4/1 -> Bus Creator3/2
  EtherCAT Async SDO Upload5/1 -> Bus Creator3/3
  Bus Creator3/1 -> Errors/1
  Saturation1/1 -> Data Type Conversion9/1
  Gain3/1 -> Sum1/1
  Constant/1 -> Sum1/2
  Data Type Conversion8/1 -> Bus Creator2/7  "in limits"
  Data Type Conversion3/1 -> Bus Creator2/8  "HW enabled"
  Data Type Conversion10/1 -> Bus Creator2/5  "quick stop"
  Data Type Conversion6/1 -> Bus Creator2/6  "switch on disable"
  Data Type Conversion11/1 -> Bus Creator2/4  "fault"
  Data Type Conversion12/1 -> Bus Creator2/3  "operation enable"
  Data Type Conversion13/1 -> Bus Creator2/2  "switched on"
  Data Type Conversion2/1 -> Bus Creator2/9  "STO selected"
  Data Type Conversion14/1 -> Bus Creator2/1  "ready to switch on"
  Control word/1 -> Data Type Conversion16/1  "control word"
  Current [mA]/1 -> Saturation1/1  "Current [mA]"

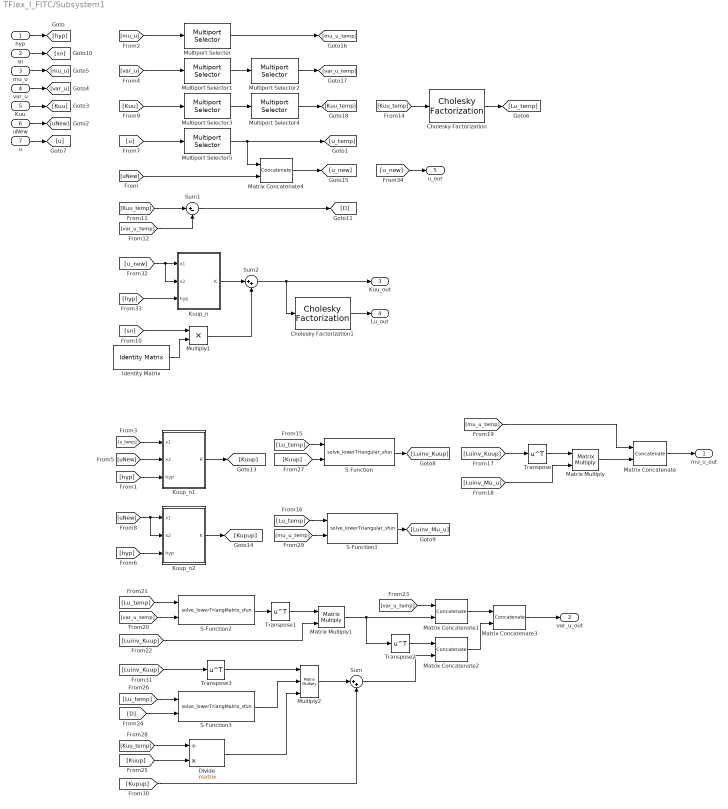
== system TFlex_I_FITC/Subsystem1 ==
  hyp : Inport
  sn : Inport  Port=2
  mu_u : Inport  Port=3
  var_u : Inport  Port=4
  Kuu : Inport  Port=5
  uNew : Inport  Port=6
  u : Inport  Port=7
  Cholesky Factorization : dspfactors/Cholesky Factorization  errmode=Warning
      settings: SourceProductName=DSP System Toolbox  SourceProductBaseCode=DS
  Cholesky Factorization1 : dspfactors/Cholesky Factorization  errmode=Warning
      settings: SourceProductName=DSP System Toolbox  SourceProductBaseCode=DS
  Divide : Product  Inputs=/*  Multiplication=Matrix(*)
  Identity Matrix : dspmtrx3/Identity Matrix  Inherit=off  N=Nkeep+1  Ts=1  dataType=double  isSigned=on  wordLen=16  udDataType=sfix(16)  fracBitsMode=Best precision  numFracBits=15  OutDataTypeStr=double  LastOutDataTypeStr=double
      settings: SourceProductName=DSP System Toolbox
  Kuup_n : MATLAB Function  TreatAsAtomicUnit=on
  Kuup_n1 : MATLAB Function  TreatAsAtomicUnit=on
  Kuup_n2 : MATLAB Function  TreatAsAtomicUnit=on
  Matrix Concatenate : Concatenate  Mode=Multidimensional array
  Matrix Concatenate1 : Concatenate  Mode=Multidimensional array  ConcatenateDimension=2
  Matrix Concatenate2 : Concatenate  Mode=Multidimensional array  ConcatenateDimension=2
  Matrix Concatenate3 : Concatenate  Mode=Multidimensional array
  Matrix Concatenate4 : Concatenate  Mode=Multidimensional array
  Matrix Multiply : Product  Multiplication=Matrix(*)
  Matrix Multiply1 : Product  Multiplication=Matrix(*)
  Multiply1 : Product
  Multiply2 : Product  Inputs=3  Multiplication=Matrix(*)
  Multiport Selector{,1,3,5} (4 alike) : dspindex/Multiport Selector  rowsOrCols=Rows  idxCellArray={ 2:Nkeep+1}  idxErrMode=Clip Index
  Multiport Selector2 : dspindex/Multiport Selector  rowsOrCols=Columns  idxCellArray={ 2:Nkeep+1}  idxErrMode=Clip Index
  Multiport Selector4 : dspindex/Multiport Selector  rowsOrCols=Columns  idxCellArray={ 2:Nkeep+1}  idxErrMode=Clip Index
  S-Function : S-Function  FunctionName=solve_lowerTriangular_sfun  Parameters=Nkeep  SFunctionDeploymentMode=off  EnableBusSupport=off
  S-Function1 : S-Function  FunctionName=solve_lowerTriangular_sfun  Parameters=Nkeep  SFunctionDeploymentMode=off  EnableBusSupport=off
  S-Function2 : S-Function  FunctionName=solve_lowerTriangMatrix_sfun  Parameters=Nkeep  SFunctionDeploymentMode=off  EnableBusSupport=off
  S-Function3 : S-Function  FunctionName=solve_lowerTriangMatrix_sfun  Parameters=Nkeep  SFunctionDeploymentMode=off  EnableBusSupport=off
  Sum : Sum  Inputs=|++
  Sum1 : Sum  Inputs=|+-
  Sum2 : Sum  Inputs=|++
  Transpose{,1..3} (4 alike) : Math  Operator=transpose  SaturateOnIntegerOverflow=on
  mu_u_out : Outport
  var_u_out : Outport  Port=2
  Kuu_out : Outport  Port=3
  Lu_out : Outport  Port=4
  u_out : Outport  Port=5
  wires:
  Kuu/1 -> [Kuu]
  uNew/1 -> [uNew]
  hyp/1 -> [hyp]
  [hyp] -> Kuup_n1/3(hyp)
  [u_temp] -> Kuup_n1/1(x1)
  [uNew] -> Kuup_n1/2(x2)
  [uNew] -> Kuup_n2/2(x2), Kuup_n2/1(x1)
  [hyp] -> Kuup_n2/3(hyp)
  var_u/1 -> [var_u]
  mu_u/1 -> [mu_u]
  Cholesky Factorization/1 -> [Lu_temp]
  [Kuu_temp] -> Cholesky Factorization/1
  [Lu_temp] -> S-Function/1
  S-Function/1 -> [Luinv_Kuup]
  S-Function1/1 -> [Luinv_Mu_u]
  [Lu_temp] -> S-Function1/1
  Kuup_n2/1(K) -> [Kupup]
  [Luinv_Kuup] -> Transpose/1
  Transpose/1 -> Matrix Multiply/1
  [Luinv_Mu_u] -> Matrix Multiply/2
  Matrix Multiply/1 -> Matrix Concatenate/2
  [mu_u_temp] -> Matrix Concatenate/1
  Matrix Concatenate/1 -> mu_u_out/1
  [var_u_temp] -> S-Function2/2
  [Lu_temp] -> S-Function2/1
  S-Function2/1 -> Transpose1/1
  Transpose1/1 -> Matrix Multiply1/1
  [Luinv_Kuup] -> Matrix Multiply1/2
  Matrix Multiply1/1 -> Matrix Concatenate1/2, Transpose2/1
  [var_u_temp] -> Matrix Concatenate1/1
  Transpose2/1 -> Matrix Concatenate2/1
  Matrix Concatenate1/1 -> Matrix Concatenate3/1
  Matrix Concatenate2/1 -> Matrix Concatenate3/2
  [D] -> S-Function3/2
  [Lu_temp] -> S-Function3/1
  [Kuup] -> Divide/2
  [Kuu_temp] -> Divide/1
  Divide/1 -> Multiply2/3
  Kuup_n1/1(K) -> [Kuup]
  [Kuup] -> S-Function/2
  [mu_u_temp] -> S-Function1/2
  [Luinv_Kuup] -> Transpose3/1
  Transpose3/1 -> Multiply2/1
  Multiply2/1 -> Sum/1
  [Kupup] -> Sum/2
  Sum/1 -> Matrix Concatenate2/2
  Matrix Concatenate3/1 -> var_u_out/1
  Identity Matrix/1 -> Multiply1/2
  [sn] -> Multiply1/1
  Matrix Concatenate4/1 -> [u_new]
  [u_new] -> Kuup_n/2(x2), Kuup_n/1(x1)
  [hyp] -> Kuup_n/3(hyp)
  Multiply1/1 -> Sum2/2
  Kuup_n/1(K) -> Sum2/1
  Sum2/1 -> Kuu_out/1, Cholesky Factorization1/1
  Cholesky Factorization1/1 -> Lu_out/1
  [u_new] -> u_out/1
  S-Function3/1 -> Multiply2/2
  Multiport Selector5/1 -> [u_temp], Matrix Concatenate4/1
  [mu_u] -> Multiport Selector/1
  Multiport Selector/1 -> [mu_u_temp]
  [var_u] -> Multiport Selector1/1
  Multiport Selector1/1 -> Multiport Selector2/1
  Multiport Selector2/1 -> [var_u_temp]
  Multiport Selector4/1 -> [Kuu_temp]
  [Kuu] -> Multiport Selector3/1
  Multiport Selector3/1 -> Multiport Selector4/1
  u/1 -> [u]
  [u] -> Multiport Selector5/1
  [uNew] -> Matrix Concatenate4/2
  sn/1 -> [sn]
  [Kuu_temp] -> Sum1/1
  [var_u_temp] -> Sum1/2
  Sum1/1 -> [D]

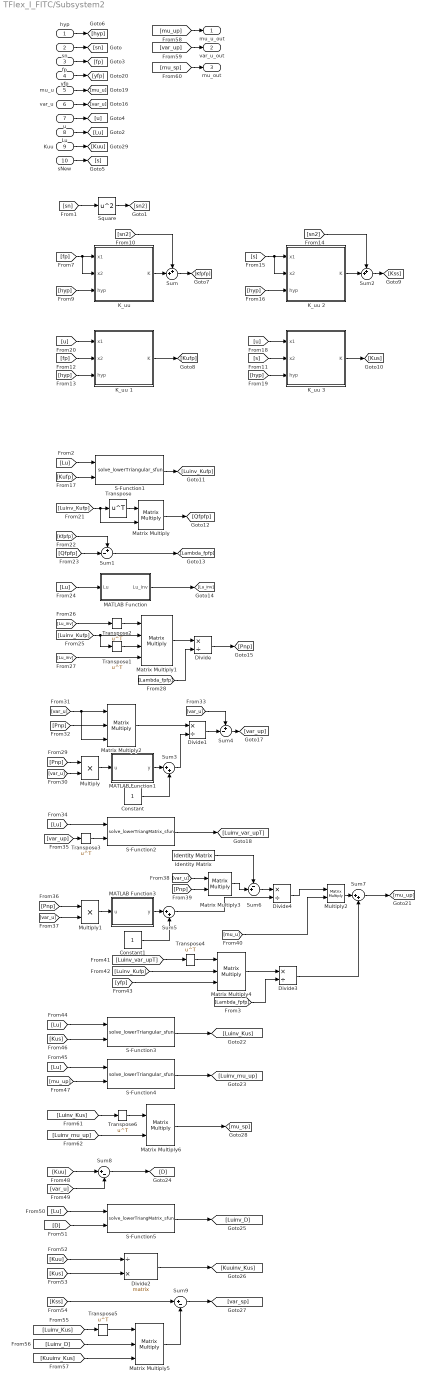
== system TFlex_I_FITC/Subsystem2 ==
  hyp : Inport
  sn : Inport  Port=2
  fp : Inport  Port=3
  yfp : Inport  Port=4
  mu_u : Inport  Port=5
  var_u : Inport  Port=6
  u : Inport  Port=7
  Lu : Inport  Port=8
  Kuu : Inport  Port=9
  sNew : Inport  Port=10
  Constant : Constant
  Constant1 : Constant
  Divide{,1,3..4} (4 alike) : Product  Inputs=*/
  Divide2 : Product  Inputs=/*  Multiplication=Matrix(*)
  Identity Matrix : dspmtrx3/Identity Matrix  Inherit=off  N=Nkeep+1  Ts=1  dataType=double  isSigned=on  wordLen=16  udDataType=sfix(16)  fracBitsMode=Best precision  numFracBits=15  OutDataTypeStr=double  LastOutDataTypeStr=double
      settings: SourceProductName=DSP System Toolbox
  "K_uu " : MATLAB Function  TreatAsAtomicUnit=on
  K_uu 1 : MATLAB Function  TreatAsAtomicUnit=on
  K_uu 2 : MATLAB Function  TreatAsAtomicUnit=on
  K_uu 3 : MATLAB Function  TreatAsAtomicUnit=on
  MATLAB Function : MATLAB Function  TreatAsAtomicUnit=on
  MATLAB Function1 : MATLAB Function  TreatAsAtomicUnit=on
  MATLAB Function3 : MATLAB Function  TreatAsAtomicUnit=on
  Matrix Multiply : Product  Multiplication=Matrix(*)
  Matrix Multiply1 : Product  Inputs=4  Multiplication=Matrix(*)
  Matrix Multiply2 : Product  Inputs=3  Multiplication=Matrix(*)
  Matrix Multiply3 : Product  Multiplication=Matrix(*)
  Matrix Multiply4 : Product  Inputs=3  Multiplication=Matrix(*)
  Matrix Multiply5 : Product  Inputs=3  Multiplication=Matrix(*)
  Matrix Multiply6 : Product  Multiplication=Matrix(*)
  Multiply : Product
  Multiply1 : Product
  Multiply2 : Product  Multiplication=Matrix(*)
  S-Function1 : S-Function  FunctionName=solve_lowerTriangular_sfun  Parameters=Nkeep+1  SFunctionDeploymentMode=off  EnableBusSupport=off
  S-Function2 : S-Function  FunctionName=solve_lowerTriangMatrix_sfun  Parameters=Nkeep+1  SFunctionDeploymentMode=off  EnableBusSupport=off
  S-Function3 : S-Function  FunctionName=solve_lowerTriangular_sfun  Parameters=Nkeep+1  SFunctionDeploymentMode=off  EnableBusSupport=off
  S-Function4 : S-Function  FunctionName=solve_lowerTriangular_sfun  Parameters=Nkeep+1  SFunctionDeploymentMode=off  EnableBusSupport=off
  S-Function5 : S-Function  FunctionName=solve_lowerTriangMatrix_sfun  Parameters=Nkeep+1  SFunctionDeploymentMode=off  EnableBusSupport=off
  Square : Math  Operator=square  SaturateOnIntegerOverflow=on
  Sum : Sum  Inputs=++|
  Sum1 : Sum  Inputs=+-|
  Sum2 : Sum  Inputs=++|
  Sum3 : Sum  Inputs=|++
  Sum4 : Sum  Inputs=+-|
  Sum5 : Sum  Inputs=|++
  Sum6 : Sum  Inputs=-+|
  Sum7 : Sum  Inputs=|++
  Sum8 : Sum  Inputs=|+-
  Sum9 : Sum  Inputs=|+-
  Transpose{,1..6} (7 alike) : Math  Operator=transpose  SaturateOnIntegerOverflow=on
  mu_u_out : Outport
  var_u_out : Outport  Port=2
  mu_out : Outport  Port=3
  wires:
  yfp/1 -> [yfp]
  sn/1 -> [sn]
  Lu/1 -> [Lu]
  var_u/1 -> [var_u]
  [sn] -> Square/1
  Square/1 -> [sn2]
  fp/1 -> [fp]
  u/1 -> [u]
  sNew/1 -> [s]
  [fp] -> "K_uu "/2(x2), "K_uu "/1(x1)
  hyp/1 -> [hyp]
  [hyp] -> "K_uu "/3(hyp)
  "K_uu "/1(K) -> Sum/2
  [sn2] -> Sum/1
  Sum/1 -> [Kfpfp]
  [fp] -> K_uu 1/2(x2)
  [hyp] -> K_uu 1/3(hyp)
  K_uu 1/1(K) -> [Kufp]
  Sum2/1 -> [Kss]
  [s] -> K_uu 2/1(x1), K_uu 2/2(x2)
  [hyp] -> K_uu 2/3(hyp)
  [sn2] -> Sum2/1
  K_uu 2/1(K) -> Sum2/2
  K_uu 3/1(K) -> [Kus]
  [u] -> K_uu 3/1(x1)
  [hyp] -> K_uu 3/3(hyp)
  [u] -> K_uu 1/1(x1)
  [s] -> K_uu 3/2(x2)
  S-Function1/1 -> [Luinv_Kufp]
  [Lu] -> S-Function1/1
  [Kufp] -> S-Function1/2
  Transpose/1 -> Matrix Multiply/1
  [Luinv_Kufp] -> Transpose/1, Matrix Multiply/2
  Matrix Multiply/1 -> [Qfpfp]
  Sum1/1 -> [Lambda_fpfp]
  [Kfpfp] -> Sum1/1
  [Qfpfp] -> Sum1/2
  [Lu] -> MATLAB Function/1(Lu)
  MATLAB Function/1(Lu_inv) -> [Lu_inv]
  [Luinv_Kufp] -> Transpose1/1, Matrix Multiply1/2
  Transpose1/1 -> Matrix Multiply1/3
  [Lu_inv] -> Transpose2/1
  Transpose2/1 -> Matrix Multiply1/1
  [Lu_inv] -> Matrix Multiply1/4
  Matrix Multiply1/1 -> Divide/1
  [Lambda_fpfp] -> Divide/2
  Divide/1 -> [Pnp]
  [Pnp] -> Multiply/1
  [var_u] -> Multiply/2
  Multiply/1 -> MATLAB Function1/1(u)
  MATLAB Function1/1(y) -> Sum3/1
  Constant/1 -> Sum3/2
  [var_u] -> Matrix Multiply2/3, Matrix Multiply2/1
  [Pnp] -> Matrix Multiply2/2
  Matrix Multiply2/1 -> Divide1/1
  Sum3/1 -> Divide1/2
  Divide1/1 -> Sum4/2
  [var_u] -> Sum4/1
  Sum4/1 -> [var_up]
  S-Function2/1 -> [Luinv_var_upT]
  [Lu] -> S-Function2/1
  [var_up] -> Transpose3/1
  Transpose3/1 -> S-Function2/2
  [var_u] -> Multiply1/2
  [Pnp] -> Multiply1/1
  Multiply1/1 -> MATLAB Function3/1(u)
  MATLAB Function3/1(y) -> Sum5/1
  Constant1/1 -> Sum5/2
  Sum5/1 -> Divide4/2
  [var_u] -> Matrix Multiply3/1
  [Pnp] -> Matrix Multiply3/2
  mu_u/1 -> [mu_u]
  Identity Matrix/1 -> Sum6/1
  Matrix Multiply3/1 -> Sum6/2
  [mu_u] -> Multiply2/2
  Transpose4/1 -> Matrix Multiply4/1
  [Luinv_var_upT] -> Transpose4/1
  [Luinv_Kufp] -> Matrix Multiply4/2
  [yfp] -> Matrix Multiply4/3
  Multiply2/1 -> Sum7/1
  Divide3/1 -> Sum7/2
  Sum7/1 -> [mu_up]
  S-Function3/1 -> [Luinv_Kus]
  S-Function4/1 -> [Luinv_mu_up]
  [Lu] -> S-Function3/1
  [Lu] -> S-Function4/1
  [Kus] -> S-Function3/2
  [mu_up] -> S-Function4/2
  [Kuu] -> Sum8/1
  [var_u] -> Sum8/2
  Sum8/1 -> [D]
  S-Function5/1 -> [Luinv_D]
  [Lu] -> S-Function5/1
  [D] -> S-Function5/2
  Divide2/1 -> [Kuuinv_Kus]
  [Kuu] -> Divide2/1
  [Kus] -> Divide2/2
  Matrix Multiply5/1 -> Sum9/2
  [Kss] -> Sum9/1
  Sum9/1 -> [var_sp]
  [Luinv_Kus] -> Transpose5/1
  Transpose5/1 -> Matrix Multiply5/1
  [Luinv_D] -> Matrix Multiply5/2
  [Kuuinv_Kus] -> Matrix Multiply5/3
  [mu_up] -> mu_u_out/1
  [var_up] -> var_u_out/1
  Transpose6/1 -> Matrix Multiply6/1
  [Luinv_Kus] -> Transpose6/1
  [Luinv_mu_up] -> Matrix Multiply6/2
  Matrix Multiply6/1 -> [mu_sp]
  [mu_sp] -> mu_out/1
  Kuu/1 -> [Kuu]
  Matrix Multiply4/1 -> Divide3/1
  [Lambda_fpfp] -> Divide3/2
  Divide4/1 -> Multiply2/1
  Sum6/1 -> Divide4/1

== system TFlex_I_FITC/Transient Setpoint Generator2 ==
  V : Inport
  Bus Creator : BusCreator  Inputs=3
  Constant : Constant  Value=r  SampleTime=ts
  Constant1 : Constant  Value=h  SampleTime=ts
  Discrete-Time Integrator : DiscreteIntegrator  gainval=1  SampleTime=ts  ICPrevOutput=DiscIntNeverNeededParam  ICPrevScaledInput=DiscIntNeverNeededParam
  Discrete-Time Integrator1 : DiscreteIntegrator  gainval=1  SampleTime=ts  ICPrevOutput=DiscIntNeverNeededParam  ICPrevScaledInput=DiscIntNeverNeededParam
  MATLAB Function2 : MATLAB Function  TreatAsAtomicUnit=on
  Scope : Scope  NumInputPorts=3
  Sum : Sum  Inputs=+-|
  Reference : Outport
  wires:
  Sum/1 -> MATLAB Function2/1(v1)
  V/1 -> Sum/2
  Constant/1 -> MATLAB Function2/3(r0)
  Constant1/1 -> MATLAB Function2/4(h0)
  Discrete-Time Integrator1/1 -> Scope/1, Bus Creator/1, Sum/1  "r"
  Discrete-Time Integrator/1 -> Discrete-Time Integrator1/1, MATLAB Function2/2(v2), Scope/2, Bus Creator/2  "r_dot"
  Bus Creator/1 -> Reference/1
  MATLAB Function2/1(output) -> Scope/3, Bus Creator/3, Discrete-Time Integrator/1  "r_ddot"

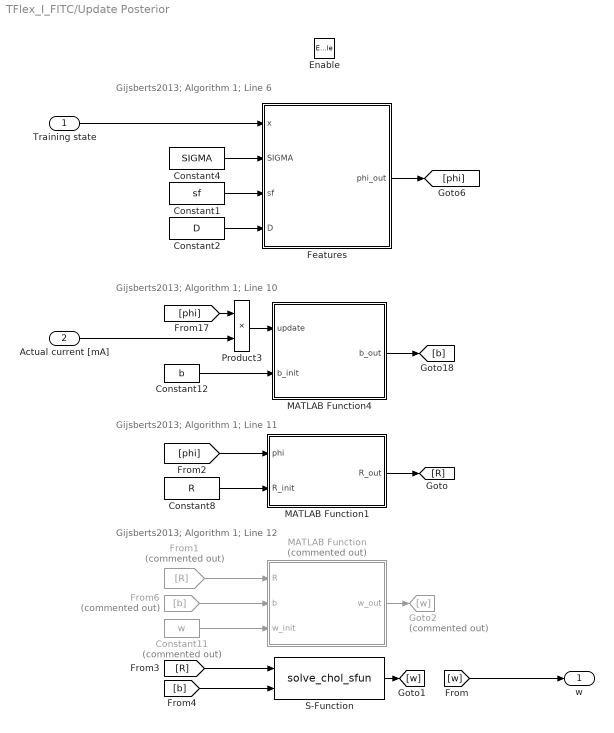
== system TFlex_I_FITC/Update Posterior ==
  note: Gijsberts2013; Algorithm 1; Line 6
  note: Gijsberts2013; Algorithm 1; Line 10
  note: Gijsberts2013; Algorithm 1; Line 11
  note: Gijsberts2013; Algorithm 1; Line 12
  Training state : Inport
  "Actual current [mA] " : Inport  Port=2
  Enable : EnablePort
  Constant1 : Constant  Value=sf  VectorParams1D=off
  Constant11 : Constant  Commented=on  Value=w  VectorParams1D=off  SampleTime=ts
  Constant12 : Constant  Value=b  VectorParams1D=off  SampleTime=ts
  Constant2 : Constant  Value=D  VectorParams1D=off
  Constant4 : Constant  Value=SIGMA  VectorParams1D=off
  Constant8 : Constant  Value=R  VectorParams1D=off  SampleTime=ts
  Features : Subsystem
  From1 : From  Commented=on  GotoTag=R
  From6 : From  Commented=on  GotoTag=b
  Goto2 : Goto  Commented=on  GotoTag=w
  MATLAB Function : MATLAB Function  Commented=on  TreatAsAtomicUnit=on
  MATLAB Function1 : MATLAB Function  TreatAsAtomicUnit=on
  MATLAB Function4 : MATLAB Function  TreatAsAtomicUnit=on
  Product3 : Product
  S-Function : S-Function  FunctionName=solve_chol_sfun  Parameters=2*D  SFunctionDeploymentMode=off  EnableBusSupport=off
  w : Outport
  wires:
  [phi] -> MATLAB Function1/1(phi)
  Training state/1 -> Features/1(x)
  Features/1(phi_out) -> [phi]
  MATLAB Function1/1(R_out) -> [R]
  Constant4/1 -> Features/2(SIGMA)
  From1/1 -> MATLAB Function/1(R)
  From6/1 -> MATLAB Function/2(b)
  Constant8/1 -> MATLAB Function1/2(R_init)
  Constant11/1 -> MATLAB Function/3(w_init)
  "Actual current [mA] "/1 -> Product3/2
  [phi] -> Product3/1
  Product3/1 -> MATLAB Function4/1(update)
  Constant12/1 -> MATLAB Function4/2(b_init)
  MATLAB Function4/1(b_out) -> [b]
  S-Function/1 -> [w]
  [w] -> w/1
  [R] -> S-Function/1
  [b] -> S-Function/2
  MATLAB Function/1(w_out) -> Goto2/1
  Constant1/1 -> Features/3(sf)
  Constant2/1 -> Features/4(D)

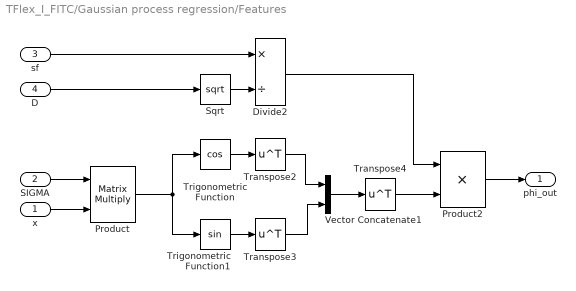
== system TFlex_I_FITC/Gaussian process regression/Features ==
  x : Inport
  SIGMA : Inport  Port=2
  sf : Inport  Port=3
  D : Inport  Port=4
  Divide2 : Product  Inputs=*/
  Product : Product  Multiplication=Matrix(*)
  Product2 : Product
  Sqrt : Sqrt  SaturateOnIntegerOverflow=on
  Transpose2 : Math  Operator=transpose  SaturateOnIntegerOverflow=on
  Transpose3 : Math  Operator=transpose  SaturateOnIntegerOverflow=on
  Transpose4 : Math  Operator=transpose  SaturateOnIntegerOverflow=on
  Trigonometric Function : Trigonometry  Operator=cos
  Trigonometric Function1 : Trigonometry
  Vector Concatenate1 : Concatenate
  phi_out : Outport
  wires:
  SIGMA/1 -> Product/1
  Product2/1 -> phi_out/1
  D/1 -> Sqrt/1
  Trigonometric Function1/1 -> Transpose3/1
  Trigonometric Function/1 -> Transpose2/1
  sf/1 -> Divide2/1
  Vector Concatenate1/1 -> Transpose4/1
  Transpose3/1 -> Vector Concatenate1/2
  Product/1 -> Trigonometric Function1/1, Trigonometric Function/1
  Divide2/1 -> Product2/1
  Transpose4/1 -> Product2/2
  Sqrt/1 -> Divide2/2
  Transpose2/1 -> Vector Concatenate1/1
  x/1 -> Product/2
